simulink model "load_tensorflow"  (R2020a)
settings: Solver=FixedStepAuto  StartTime=0.0  StopTime=inf  FixedStep=0.05  RelTol=1e-3
libraries: robotlib x5
settings Model: Creator=ivory  LastModifiedBy=ivory
settings OptimizationCC: EnhancedBackFolding=on  PassReuseOutputArgsAs=Individual arguments  ZeroExternalMemoryAtStartup=off  ZeroInternalMemoryAtStartup=off  MaxStackSize=64  OptimizeBlockOrder=speed  DifferentSizesBufferReuse=on  OptimizationCustomize=off  EfficientTunableParamExpr=on
settings DebuggingCC: ParameterTunabilityLossMsg=error
settings HardwareCC: ProdBitPerPointer=32  ProdBitPerSizeT=32  ProdBitPerPtrDiffT=32  ProdLargestAtomicFloat=None  ProdIntDivRoundTo=Undefined  ProdEndianess=Unspecified  ProdWordSize=32  ProdHWDeviceType=Generic->Unspecified (assume 32-bit Generic)
settings SFSimCC: MATLABDynamicMemAlloc=off
settings RTWCC: SystemTargetFile=ert.tlc  HardwareBoard=Robot Operating System (ROS)  TemplateMakefile=ert_default_tmf  Toolchain=Catkin  TargetLang=C++
settings CodeAppCC: ForceParamTrailComments=on  IgnoreCustomStorageClasses=off  OperatorAnnotations=on  SimulinkDataObjDesc=on  SFDataObjDesc=on  InsertBlockDesc=on

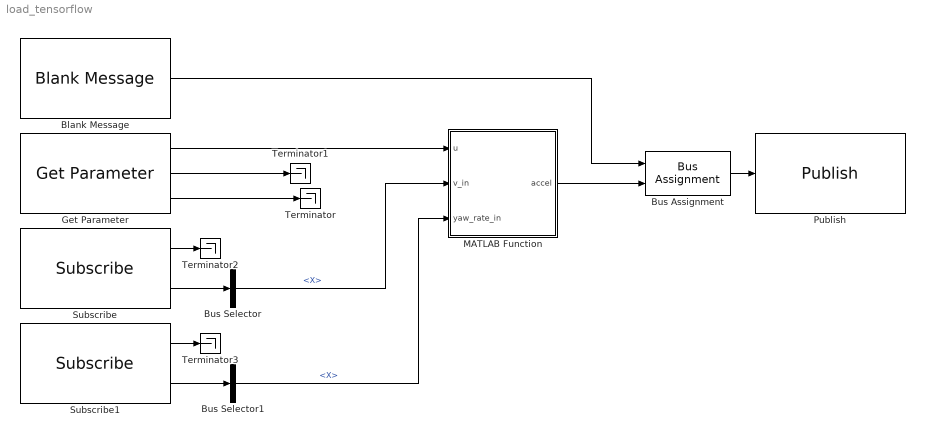
== system load_tensorflow ==
  Blank Message : robotlib/Blank Message  messageClass=Message  entityType=geometry_msgs/Twist  messageType=geometry_msgs/Twist  SampleTime=inf
  Bus Assignment : BusAssignment  AssignedSignals=Linear.X
  Bus Selector : BusSelector  OutputSignals=Linear.X
  Bus Selector1 : BusSelector  OutputSignals=Linear.X
  Get Parameter : robotlib/Get Parameter  ParameterSource=Specify your own  ParameterName=model_path  ParameterType=uint8[] (string)  ParameterMaxArrayLength=256  ParameterInitialValue=0  SampleTime=-1  ShowErrorCodeOutput=on  ModelName=load_tensorflow  BlockId=ParamGet_load_tensorflow_1
      settings: SourceProductBaseCode=RR
  MATLAB Function : MATLAB Function  TreatAsAtomicUnit=on
  Publish : robotlib/Publish  topicSource=Specify your own  topic=accel  messageType=geometry_msgs/Twist  messageQueueLength=1
  Subscribe : robotlib/Subscribe  topicSource=Specify your own  topic=cmd_vel  messageType=geometry_msgs/Twist  sampleTime=-1  messageQueueLength=1
  Subscribe1 : robotlib/Subscribe  topicSource=Specify your own  topic=yaw_rate  messageType=geometry_msgs/Twist  sampleTime=-1  messageQueueLength=1
  Terminator{,1..3} (4 alike) : Terminator
  wires:
  Get Parameter/3 -> Terminator/1
  Get Parameter/1 -> MATLAB Function/1(u)
  Get Parameter/2 -> Terminator1/1
  Subscribe/1 -> Terminator2/1
  Subscribe/2 -> Bus Selector/1
  Bus Selector/1 -> MATLAB Function/2(v_in)  "<X>"
  Subscribe1/2 -> Bus Selector1/1
  Subscribe1/1 -> Terminator3/1
  Bus Selector1/1 -> MATLAB Function/3(yaw_rate_in)  "<X>"
  Blank Message/1 -> Bus Assignment/1
  MATLAB Function/1(accel) -> Bus Assignment/2
  Bus Assignment/1 -> Publish/1

== matlab function load_tensorflow/MATLAB Function ==
  data: u input; v_in input; yaw_rate_in input; accel output
function accel = fcn(u, v_in, yaw_rate_in)

layer = importKerasLayers(u, 'OutputLayerType','regression');
lgraph = layerGraph(layer);
layer_last = regressionLayer('Name','routput');
lgraph = replaceLayer(lgraph,findPlaceholderLayers(layer)',layer_last);
net = assembleNetwork(lgraph);
accel = net.predict([v_in, yaw_rate_in]);

end
